simulink model "peak_current_mode_3phase"  (R2021b)
settings: Solver=VariableStepAuto  StartTime=0.0  StopTime=10  RelTol=1e-3
libraries: spsCurrentMeasurementLib x1, spsDCMachineLib x1, spsDCVoltageSourceLib x1, spsThreePhaseVIMeasurementLib x1, spsThreePhaseSourceLib x1, spsUniversalBridgeLib x1, spsVoltageMeasurementLib x1, spspowerguiLib x1
settings Model: Creator=Göktuğ  LastModifiedBy=Göktuğ

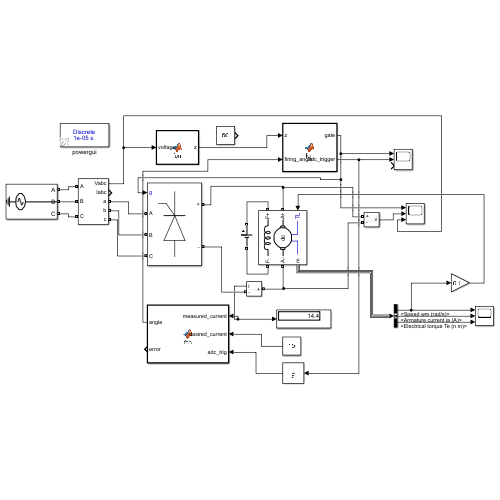
[thumbnail: Simulink's stored preview of the top-level diagram]
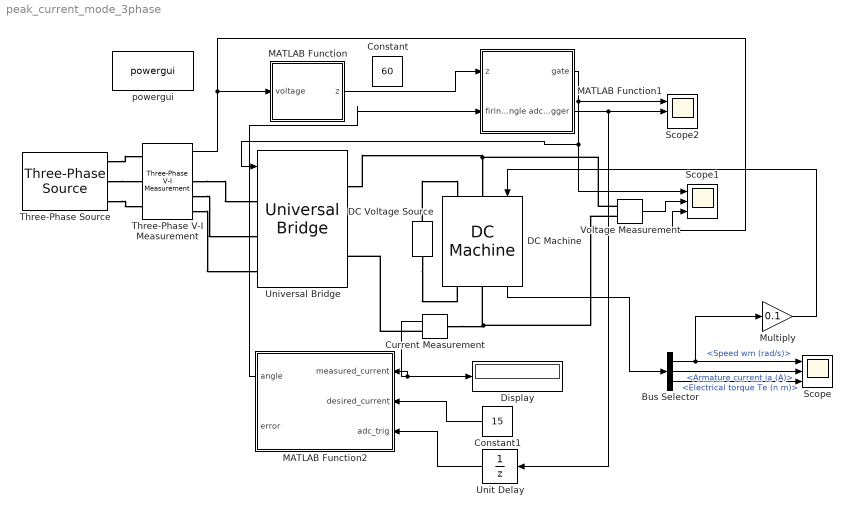
== system peak_current_mode_3phase ==
  Bus Selector : BusSelector  OutputSignals=Speed wm (rad/s),Armature current ia (A),Electrical torque Te (n m)
  Constant : Constant  Value=60
  Constant1 : Constant  Value=15
  Current Measurement : spsCurrentMeasurementLib/Current Measurement  PhasorSimulation=off  OutputType=Complex  PSBequivalent=0
  DC Machine : spsDCMachineLib/DC Machine  PresetModel=No  MechanicalLoad=Torque TL  FieldType=Wound  ShowDetailedParameters=on  MeasurementBus=off  RLa="[ 0.8  12.5e-3]"  RLf="[ 240  120]"  Laf=1.8  MachineConstant=Torque constant (N.m/A)  Ke=1.8  Kt=1.8  J=1  Bm=0  Tf=0  w0=0  Ifinit=0.625  TsPowergui=0  TsBlock=-1
  DC Voltage Source : spsDCVoltageSourceLib/DC Voltage Source  Amplitude=150  Measurements=None
  Display : Display
  MATLAB Function : MATLAB Function  TreatAsAtomicUnit=on
  MATLAB Function1 : MATLAB Function  TreatAsAtomicUnit=on
  MATLAB Function2 : MATLAB Function  TreatAsAtomicUnit=on
  Multiply : Gain  Gain=0.1
  Scope : Scope  NumInputPorts=3
  Scope1 : Scope  NumInputPorts=3
  Scope2 : Scope  NumInputPorts=3
  Three-Phase V-I Measurement : spsThreePhaseVIMeasurementLib/Three-Phase V-I Measurement  VoltageMeasurement=phase-to-ground  SetLabelV=off  LabelV=Vabc  Vpu=off  VpuLL=off  CurrentMeasurement=yes  SetLabelI=off  LabelI=Iabc  Ipu=off  Pbase=100e6  Vbase=500e3  OutputType=Complex  PhasorSimulation=off  PSBequivalent=0
  Three-Phase Source : spsThreePhaseSourceLib/Three-Phase Source  InternalConnection=Yg  VoltagePhases=off  Voltage=180  PhaseAngle=0  Voltage_phases=[25e3 25e3 25e3]/sqrt(3)  PhaseAngles_phases=[0 -120 +120]  Frequency=50  NonIdealSource=on  SpecifyImpedance=off  Resistance=0  Inductance=0  ShortCircuitLevel=100e6  BaseVoltage=0  XRratio=7  BusType=swing  Pref=10e3  Qref=0  Prefabc=[10e3, 10e3, 10e3]  Qrefabc=[0, 0, 0]  Qmin=-inf  Qmax=inf
  Unit Delay : UnitDelay  SampleTime=-1  HasFrameUpgradeWarning=on
  Universal Bridge : spsUniversalBridgeLib/Universal Bridge  Arms=3  SnubberResistance=1e5  SnubberCapacitance=inf  Device=Thyristors  Ron=1e-3  Lon=0  ForwardVoltages="[  0  0  ]"  ForwardVoltage=0  GTOparameters=[ 10e-6 , 20e-6 ]  IGBTparameters=[ 1e-6 , 2e-6 ]  Measurements=None  Measurements_2=None  converterType=Rectifier
  Voltage Measurement : spsVoltageMeasurementLib/Voltage Measurement  PhasorSimulation=off  OutputType=Complex  PSBequivalent=0
  powergui : spspowerguiLib/powergui  Priority=1  SimulationMode=Discrete  SampleTime=10e-6  frequency=60  Iterations=50  frequencyindice=0  Pbase=100e6  ErrMax=1e-4  UnitsV=kV  UnitsW=MW  buscounter=0  FunctionMessages=off  echomessages=off  EnableUseOfTLC=off  CurrentSourceSwitches=off  DisableSnubberDevices=off  DisableRonSwitches=off  DisableVfSwitches=off  DisplayEquations=off  AutomaticDiscreteSolvers=off  SolverType=Tustin/Backward Euler (TBE)  Interpol=off  ExternalGateDelay=off  methode=off  Ts=100  x0status=blocks  SPID=on  SwTol=0  HookPort=off  NonlinearTolerance=1e-4  nMaxIteration=100  ContinueOnMaxIteration=off  RestoreLinks=warning  ResistiveCurrentMeasurement=off  Frange=[0:2:500]  Ylog=off  Xlog=on  ShowGrid=off  save=off  variable=ZData  structure=0  ZoomFFT=off  StartTime=0.0  cycles=1  DisplayStyle=1  fundamental=60  FreqAxis=off  MaxFrequency=1000  frequencyindicesteady=1  RmsSteady=1  display=off
  wires:
  MATLAB Function/1(z) -> MATLAB Function1/1(z)
  MATLAB Function1/1(gate) -> Scope2/1, Universal Bridge/1, Scope1/1
  Voltage Measurement/1 -> Scope1/2
  Three-Phase V-I Measurement/1 -> Scope1/3, MATLAB Function/1(voltage)
  Current Measurement/1 -> Display/1, MATLAB Function2/1(measured_current)
  Constant1/1 -> MATLAB Function2/2(desired_current)
  MATLAB Function2/1(angle) -> MATLAB Function1/2(firing_angle)
  DC Machine/1 -> Bus Selector/1
  Bus Selector/1 -> Multiply/1, Scope/1  "<Speed wm (rad/s)>"
  Bus Selector/2 -> Scope/2  "<Armature current ia (A)>"
  Bus Selector/3 -> Scope/3  "<Electrical torque Te (n m)>"
  Multiply/1 -> DC Machine/1
  MATLAB Function1/2(adc_trigger) -> Unit Delay/1, Scope2/2
  Unit Delay/1 -> MATLAB Function2/3(adc_trig)
  connections:
  Three-Phase Source/RConn1 -- Three-Phase V-I Measurement/LConn1
  Three-Phase Source/RConn2 -- Three-Phase V-I Measurement/LConn2
  Three-Phase Source/RConn3 -- Three-Phase V-I Measurement/LConn3
  Three-Phase V-I Measurement/RConn1 -- Universal Bridge/LConn1
  Three-Phase V-I Measurement/RConn2 -- Universal Bridge/LConn2
  Three-Phase V-I Measurement/RConn3 -- Universal Bridge/LConn3
  DC Voltage Source/RConn1 -- DC Machine/LConn2
  DC Voltage Source/LConn1 -- DC Machine/RConn2
  Universal Bridge/RConn1 -- Voltage Measurement/LConn1 -- DC Machine/LConn1
  Voltage Measurement/LConn2 -- Current Measurement/LConn1 -- DC Machine/RConn1
  Current Measurement/RConn1 -- Universal Bridge/RConn2

== matlab function peak_current_mode_3phase/MATLAB Function1 ==
  data: z input; gate output size=[1 6]; firing_angle input; adc_trigger output
function [gate, adc_trigger]= fcn(z, firing_angle)

persistent angle_pA;

persistent step;

if isempty(step)
    step = 6;
end

if isempty(angle_pA)
    angle_pA = 0;
end

d2r=pi/180;
r2d=180/pi;


if z==1 %sync first phase
    angle_pA = 0;
else
    angle_pA = angle_pA + 0.18;
end

%bridge config is 1 3 5
%                 4 6 2

if(r2d*angdiff((firing_angle+30)*d2r,angle_pA*d2r)>=0 && r2d*angdiff((firing_angle+90)*d2r,angle_pA*d2r)<0)%step1
    step = 1;
    gate_sig = [1 0 0 0 0 0];
elseif(r2d*angdiff((firing_angle+90)*d2r,angle_pA*d2r)>=0 && r2d*angdiff((firing_angle+150)*d2r,angle_pA*d2r)<0)%step2
    step = 2;
    gate_sig = [0 1 0 0 0 0];
elseif(r2d*angdiff((firing_angle+150)*d2r,angle_pA*d2r)>=0 && r2d*angdiff((firing_angle+210)*d2r,angle_pA*d2r)<0)%step3
    step = 3;
    gate_sig = [0 0 1 0 0 0];
elseif(r2d*angdiff((firing_angle+210)*d2r,angle_pA*d2r)>=0 && r2d*angdiff((firing_angle+270)*d2r,angle_pA*d2r)<0)%step4
    step = 4;
    gate_sig = [0 0 0 1 0 0];
elseif(r2d*angdiff((firing_angle+270)*d2r,angle_pA*d2r)>=0 && r2d*angdiff((firing_angle+330)*d2r,angle_pA*d2r)<0)%step5
    step = 5;
    gate_sig = [0 0 0 0 1 0];
elseif(r2d*angdiff((firing_angle+330)*d2r,angle_pA*d2r)>=0 && r2d*angdiff((firing_angle+30)*d2r,angle_pA*d2r)<0)%step6
    step = 6;
    gate_sig = [0 0 0 0 0 1];
else
    gate_sig = [0 0 0 0 0 0];
end
if(r2d*angdiff((firing_angle+59.5)*d2r,angle_pA*d2r)>=0 && r2d*angdiff((firing_angle+60.5)*d2r,angle_pA*d2r)<0)%step1
    adc = 1;
elseif(r2d*angdiff((firing_angle+119.5)*d2r,angle_pA*d2r)>=0 && r2d*angdiff((firing_angle+120.5)*d2r,angle_pA*d2r)<0)%step2
    adc = 1;
elseif(r2d*angdiff((firing_angle+179.5)*d2r,angle_pA*d2r)>=0 && r2d*angdiff((firing_angle+180.5)*d2r,angle_pA*d2r)<0)%step3
    adc = 1;
elseif(r2d*angdiff((firing_angle+239.5)*d2r,angle_pA*d2r)>=0 && r2d*angdiff((firing_angle+240.5)*d2r,angle_pA*d2r)<0)%step4
    adc = 1;
elseif(r2d*angdiff((firing_angle+300.5)*d2r,angle_pA*d2r)>=0 && r2d*angdiff((firing_angle+301.5)*d2r,angle_pA*d2r)<0)%step5
    adc = 1;
elseif(r2d*angdiff((firing_angle+359.5)*d2r,angle_pA*d2r)>=0 && r2d*angdiff((firing_angle+0.5)*d2r,angle_pA*d2r)<0)%step6
    adc = 1;
else
    adc = 0;
end
gate = gate_sig;
adc_trigger = adc;
end

== matlab function peak_current_mode_3phase/MATLAB Function ==
  data: voltage input; z output
function z   = fcn( voltage)
    
    persistent past_voltage;
    
    if isempty(past_voltage)
        past_voltage = 0;
    end

    if(past_voltage < 0 && voltage(1)>=0)
        z=1;
    else
        z=0;
    end
    past_voltage = voltage(1);
end

== matlab function peak_current_mode_3phase/MATLAB Function2 ==
  data: measured_current input; desired_current input; angle output; error output; adc_trig input
function [angle, error]= fcn(measured_current,desired_current, adc_trig)
persistent firing_angle;


if(isempty(firing_angle))
    firing_angle = 120;
end

%lets make a cheat, we know that our sample time, 10uS, for one step we need 20mS/6 time which is 3.33mS and app 333step call for our function
%why we are making cheat? because i dont know how to sync the
%measurements, in current configration we are makking measurements in
%random times. This means that we have to somehow, calculate it mean value
%or rms value. Making it causes unnecessary computation, lets assume that
%inductor current is triangular wave and take the middle point as 167.
%measurement. Then by using only every 167. measurement we can calculate
%the current, but this causes a problem. Depending on the firing angle
%actually this number should move. (In a mcu it is just a timer trick but
%in matlab it is really complicated for me) So my last decision is adding
%an adc trigger input, i will create the trigger using firing angle block
%and when it is 1 i will calculate the next firing angle.
if(adc_trig == 1)
    if(desired_current>measured_current)
        firing_angle = firing_angle - 0.05;
    elseif(measured_current>desired_current)
        firing_angle = firing_angle + 0.05;
    end
    if(firing_angle<0)
        firing_angle = 0;
    elseif(firing_angle>120)
        firing_angle=120;
    end

end
    error = desired_current - measured_current;
    angle = firing_angle;
end
